simulink model "M002_SOFC_meca"  (R2021a)
settings: Solver=VariableStepAuto  StartTime=0.0  StopTime=1037  RelTol=1e-3
values from neighbouring files (symbols this model uses):
  p = SOFC_p    [M002_init_SOFC_meca.m]
  x0_SOFC = SOFC_init    [M002_init_SOFC_meca.m]
undefined symbols (not defined in the file or in its folder): nearst_p
settings Model: Creator=djoroya  LastModifiedBy=djoroya

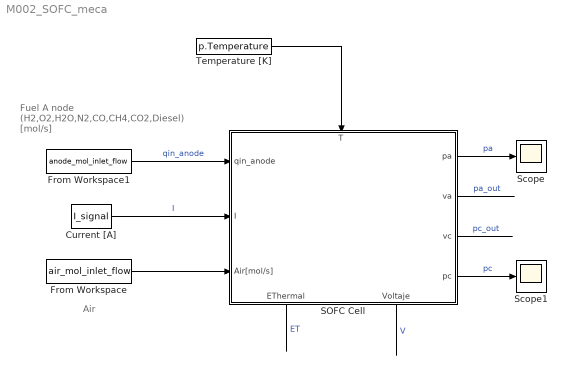
== system M002_SOFC_meca ==
  note: Fuel
      | A node
      | (H2,O2,H2O,N2,CO,CH4,CO2,Diesel)
      | [mol/s]
  note: Air
  Current [A] : FromWorkspace  VariableName=I_signal
  From Workspace : FromWorkspace  VariableName=air_mol_inlet_flow
  From Workspace1 : FromWorkspace  VariableName=anode_mol_inlet_flow
  SOFC Cell : Subsystem  mask{p=p, x0=x0_SOFC}
      mask prompts: p "params"
      settings: PortSchema="{\"entries\":[{\"content\":{\"sides\":[{\"content\":{\"connectorIds\":[\"In1\",\"In2\",\"In3\"]},\"type\":\"ConnectorPlacement.EquallySpacedRectSide\",\"uuid\":\"6cca8e4f-6db2-48de-a60a-b6fbc16877c6\"},{\"content\":{\"connectorIds\":[\"Out1\",\"Out2\",\"Out3\",\"Out4\"],\"side\":\"RIGHT\"},\"type\":\"ConnectorPlacement.EquallySpacedRectSide\",\"uuid\":\"c481f6d1-531d-4215-9ae0-5807376c0625\"},{\"content\":{\"connectorIds\":[\"In4\"],\"side\":\"TOP\"},\"type\":\"ConnectorPlacement.EquallySpacedRectSide\",\"uuid\":\"76720726-927e-4340-b17d-e33f4db2c782\"},{\"content\":{\"connectorIds\":[\"Out5\",\"Out6\"],\"side\":\"BOTTOM\"},\"type\":\"ConnectorPlacement.EquallySpacedRectSide\",\"uuid\":\"7ed108e3-6588-44d6-8f3d-9789ffe258a7\"}]},\"type\":\"ConnectorPlacement.EquallySpacedConnector\",\"uuid\":\"f9228f26-0840-43d6-932a-2fdb8a27bf20\"}],\"packageUris\":[\"http://schema.mathworks.com/mf0/Connector/R2020b\"],\"version\":\"1.0\"}"
  Scope : Scope
  Scope1 : Scope
  Temperature [K] : Constant  Value=p.Temperature
  wires:
  From Workspace1/1 -> SOFC Cell/1(qin_anode)  "qin_anode"
  Current [A]/1 -> SOFC Cell/2(I)  "I"
  Temperature [K]/1 -> SOFC Cell/4(T)
  From Workspace/1 -> SOFC Cell/3(Air[mol/s])
  SOFC Cell/1(pa) -> Scope/1  "pa"
  SOFC Cell/4(pc) -> Scope1/1  "pc"
  SOFC Cell/2(va) -> ?  "pa_out"
  SOFC Cell/3(vc) -> ?  "pc_out"
  SOFC Cell/5(EThermal) -> ?  "ET"
  SOFC Cell/6(Voltaje) -> ?  "V"

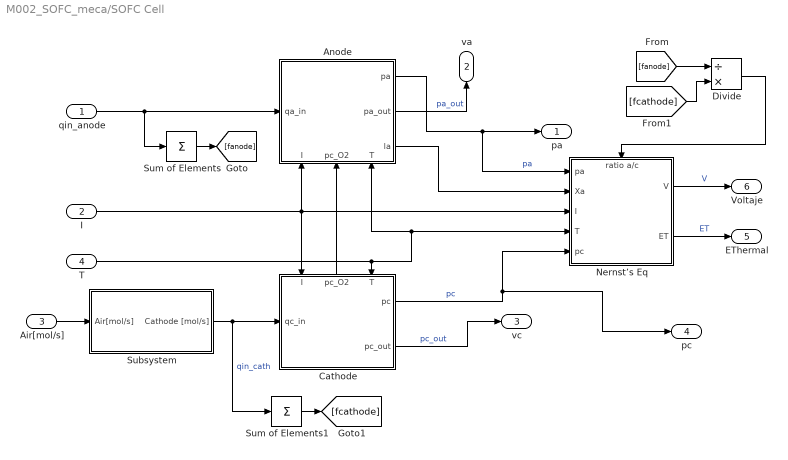
== system M002_SOFC_meca/SOFC Cell ==
  qin_anode : Inport
  I : Inport  Port=2
  Air[mol/s] : Inport  Port=3
  T : Inport  Port=4
  Anode : Subsystem
      settings: PortSchema="{\"entries\":[{\"content\":{\"sides\":[{\"content\":{\"connectorIds\":[\"In1\"]},\"type\":\"ConnectorPlacement.EquallySpacedRectSide\",\"uuid\":\"1d27f661-9cb9-482d-ac43-89e84d52643b\"},{\"content\":{\"connectorIds\":[\"Out1\",\"Out2\",\"Out3\"],\"side\":\"RIGHT\"},\"type\":\"ConnectorPlacement.EquallySpacedRectSide\",\"uuid\":\"62ac897d-5819-4e9c-a19f-e210851aefa2\"},{\"content\":{\"connectorIds\":[],\"side\":\"TOP\"},\"type\":\"ConnectorPlacement.EquallySpacedRectSide\",\"uuid\":\"1380e9d4-c5ac-42ce-b6fc-00336cc8edba\"},{\"content\":{\"connectorIds\":[\"In2\",\"In3\",\"In4\"],\"side\":\"BOTTOM\"},\"type\":\"ConnectorPlacement.EquallySpacedRectSide\",\"uuid\":\"0e36fd1a-38eb-48cb-8834-06d558b43614\"}]},\"type\":\"ConnectorPlacement.EquallySpacedConnector\",\"uuid\":\"79a72313-dbdc-4de5-b88f-787bafe984c7\"}],\"packageUris\":[\"http://schema.mathworks.com/mf0/Connector/R2020b\"],\"version\":\"1.0\"}"
  Cathode : Subsystem
      settings: PortSchema="{\"entries\":[{\"content\":{\"sides\":[{\"content\":{\"connectorIds\":[\"In1\"]},\"type\":\"ConnectorPlacement.EquallySpacedRectSide\",\"uuid\":\"1d27f661-9cb9-482d-ac43-89e84d52643b\"},{\"content\":{\"connectorIds\":[\"Out1\",\"Out2\"],\"side\":\"RIGHT\"},\"type\":\"ConnectorPlacement.EquallySpacedRectSide\",\"uuid\":\"62ac897d-5819-4e9c-a19f-e210851aefa2\"},{\"content\":{\"connectorIds\":[\"In2\",\"Out3\",\"In3\"],\"side\":\"TOP\"},\"type\":\"ConnectorPlacement.EquallySpacedRectSide\",\"uuid\":\"1380e9d4-c5ac-42ce-b6fc-00336cc8edba\"}]},\"type\":\"ConnectorPlacement.EquallySpacedConnector\",\"uuid\":\"79a72313-dbdc-4de5-b88f-787bafe984c7\"}],\"packageUris\":[\"http://schema.mathworks.com/mf0/Connector/R2020b\"],\"version\":\"1.0\"}"
  Divide : Product  Inputs=/*
  "Nernst’s Eq " : Subsystem
      settings: PortSchema="{\"entries\":[{\"content\":{\"sides\":[{\"content\":{\"connectorIds\":[\"In1\",\"In2\",\"In3\",\"In4\",\"In5\"]},\"type\":\"ConnectorPlacement.EquallySpacedRectSide\",\"uuid\":\"1b300774-e64d-4a8a-a2e9-ecdc71723fee\"},{\"content\":{\"connectorIds\":[\"Out1\",\"Out2\"],\"side\":\"RIGHT\"},\"type\":\"ConnectorPlacement.EquallySpacedRectSide\",\"uuid\":\"354a04f1-cc66-4a63-8c50-8080316e29e9\"},{\"content\":{\"connectorIds\":[\"In6\"],\"side\":\"TOP\"},\"type\":\"ConnectorPlacement.EquallySpacedRectSide\",\"uuid\":\"b48b7bda-dd37-468f-ab7d-ccd563a69f0b\"}]},\"type\":\"ConnectorPlacement.EquallySpacedConnector\",\"uuid\":\"ddfd4041-6e53-4893-9028-34e5ff9f82d6\"}],\"packageUris\":[\"http://schema.mathworks.com/mf0/Connector/R2020b\"],\"version\":\"1.0\"}"
  Subsystem : Subsystem
  Sum of Elements : Sum  Inputs=+
  Sum of Elements1 : Sum  Inputs=+
  pa : Outport
  va : Outport  Port=2
  vc : Outport  Port=3
  pc : Outport  Port=4
  EThermal : Outport  Port=5
  Voltaje : Outport  Port=6
  wires:
  Air[mol/s]/1 -> Subsystem/1(Air[mol/s])
  Anode/1(pa) -> pa/1, "Nernst’s Eq "/1(pa)  "pa"
  Anode/2(pa_out) -> va/1  "pa_out"
  Cathode/1(pc) -> pc/1, "Nernst’s Eq "/5(pc)  "pc"
  Subsystem/1(Cathode [mol/s]) -> Sum of Elements1/1, Cathode/1(qc_in)  "qin_cath"
  "Nernst’s Eq "/2(ET) -> EThermal/1  "ET"
  Cathode/3(pc_O2) -> Anode/3(pc_O2)
  Cathode/2(pc_out) -> vc/1  "pc_out"
  I/1 -> Cathode/2(I), "Nernst’s Eq "/3(I), Anode/2(I)
  T/1 -> "Nernst’s Eq "/4(T), Anode/4(T), Cathode/3(T)
  qin_anode/1 -> Anode/1(qa_in), Sum of Elements/1
  "Nernst’s Eq "/1(V) -> Voltaje/1  "V"
  Anode/3(la) -> "Nernst’s Eq "/2(Xa)
  Sum of Elements/1 -> [fanode]
  Sum of Elements1/1 -> [fcathode]
  [fanode] -> Divide/1
  [fcathode] -> Divide/2
  Divide/1 -> "Nernst’s Eq "/6(ratio a/c)

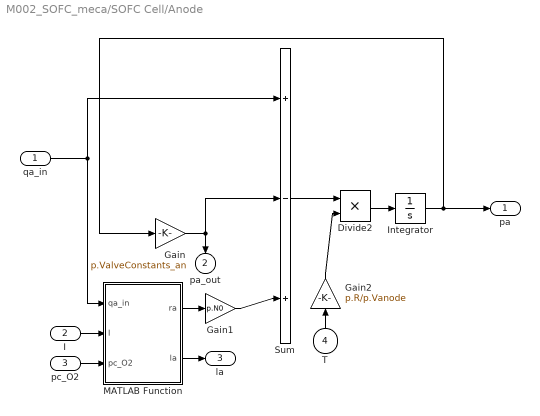
== system M002_SOFC_meca/SOFC Cell/Anode ==
  qa_in : Inport
  I : Inport  Port=2
  pc_O2 : Inport  Port=3
  T : Inport  Port=4
  Divide2 : Product  Inputs=**
  Gain : Gain  Gain=p.ValveConstants_an
  Gain1 : Gain  Gain=p.N0
  Gain2 : Gain  Gain=p.R/p.Vanode
  Integrator : Integrator  InitialCondition=x0_SOFC.pa
  MATLAB Function : MATLAB Function  TreatAsAtomicUnit=on
  Sum : Sum  Inputs=|+-+
  pa : Outport
  pa_out : Outport  Port=2
  la : Outport  Port=3
  wires:
  Sum/1 -> Divide2/1
  Integrator/1 -> pa/1, Gain/1
  Gain2/1 -> Divide2/2
  qa_in/1 -> Sum/1, MATLAB Function/1(qa_in)
  Divide2/1 -> Integrator/1
  Gain/1 -> pa_out/1, Sum/2
  I/1 -> MATLAB Function/2(I)
  T/1 -> Gain2/1
  MATLAB Function/2(la) -> la/1
  pc_O2/1 -> MATLAB Function/3(pc_O2)
  MATLAB Function/1(ra) -> Gain1/1
  Gain1/1 -> Sum/3

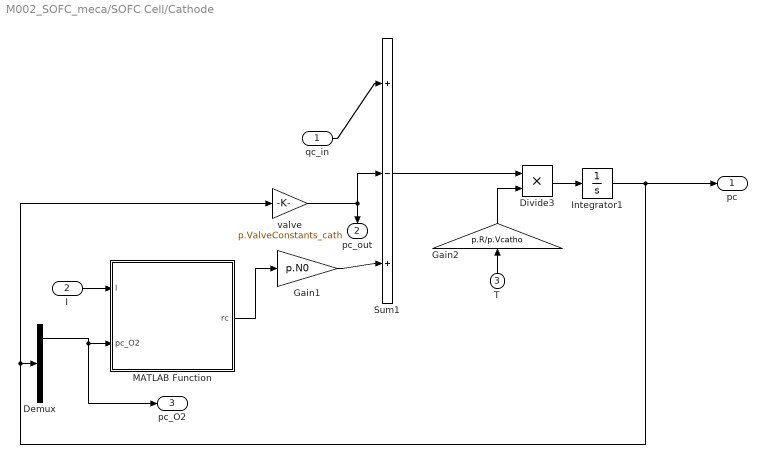
== system M002_SOFC_meca/SOFC Cell/Cathode ==
  qc_in : Inport
  I : Inport  Port=2
  T : Inport  Port=3
  Demux : Demux  Outputs=8
  Divide3 : Product  Inputs=**
  Gain1 : Gain  Gain=p.N0
  Gain2 : Gain  Gain=p.R/p.Vcatho
  Integrator1 : Integrator  InitialCondition=x0_SOFC.pc
  MATLAB Function : MATLAB Function  TreatAsAtomicUnit=on
  Sum1 : Sum  Inputs=|+-+
  valve : Gain  Gain=p.ValveConstants_cath
  pc : Outport
  pc_out : Outport  Port=2
  pc_O2 : Outport  Port=3
  wires:
  Sum1/1 -> Divide3/1
  Integrator1/1 -> valve/1, Demux/1, pc/1
  Divide3/1 -> Integrator1/1
  qc_in/1 -> Sum1/1
  Gain2/1 -> Divide3/2
  T/1 -> Gain2/1
  valve/1 -> pc_out/1, Sum1/2
  I/1 -> MATLAB Function/1(I)
  Demux/2 -> pc_O2/1, MATLAB Function/2(pc_O2)
  MATLAB Function/1(rc) -> Gain1/1
  Gain1/1 -> Sum1/3

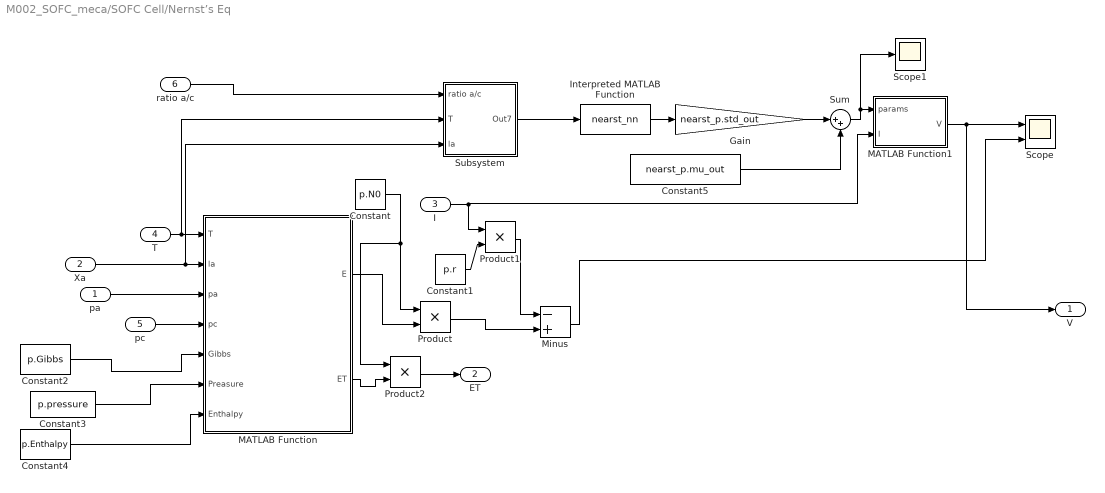
== system M002_SOFC_meca/SOFC Cell/Nernst’s Eq  ==
  pa : Inport
  Xa : Inport  Port=2
  I : Inport  Port=3
  T : Inport  Port=4
  pc : Inport  Port=5
  ratio a/c : Inport  Port=6
  Constant : Constant  Value=p.N0
  Constant1 : Constant  Value=p.r
  Constant2 : Constant  Value=p.Gibbs  OutDataTypeStr=Bus:slBus1
  Constant3 : Constant  Value=p.pressure
  Constant4 : Constant  Value=p.Enthalpy  OutDataTypeStr=Bus:slBus1
  Constant5 : Constant  Value=nearst_p.mu_out
  Gain : Gain  Gain=nearst_p.std_out
  Interpreted MATLAB Function : MATLABFcn  MATLABFcn=nearst_nn
  MATLAB Function : MATLAB Function  TreatAsAtomicUnit=on
  MATLAB Function1 : MATLAB Function  TreatAsAtomicUnit=on
  Minus : Sum  Inputs=-+
  Product : Product
  Product1 : Product
  Product2 : Product
  Scope : Scope  NumInputPorts=2
  Scope1 : Scope
  Subsystem : Subsystem
  Sum : Sum  Inputs=|++
  V : Outport
  ET : Outport  Port=2
  wires:
  MATLAB Function/1(E) -> Product/2
  Constant/1 -> Product2/1, Product/1
  I/1 -> Product1/1, MATLAB Function1/2(I)
  Constant1/1 -> Product1/2
  Product/1 -> Minus/2
  Minus/1 -> Scope/2
  Product1/1 -> Minus/1
  pa/1 -> MATLAB Function/3(pa)
  pc/1 -> MATLAB Function/4(pc)
  Constant2/1 -> MATLAB Function/5(Gibbs)
  T/1 -> Subsystem/2(T), MATLAB Function/1(T)
  Xa/1 -> Subsystem/3(la), MATLAB Function/2(la)
  Constant3/1 -> MATLAB Function/6(Preasure)
  Constant4/1 -> MATLAB Function/7(Enthalpy)
  Product2/1 -> ET/1
  MATLAB Function/2(ET) -> Product2/2
  ratio a/c/1 -> Subsystem/1(ratio a/c)
  Subsystem/1(Out7) -> Interpreted MATLAB Function/1
  Interpreted MATLAB Function/1 -> Gain/1
  Gain/1 -> Sum/1
  Constant5/1 -> Sum/2
  Sum/1 -> Scope1/1, MATLAB Function1/1(params)
  MATLAB Function1/1(V) -> V/1, Scope/1

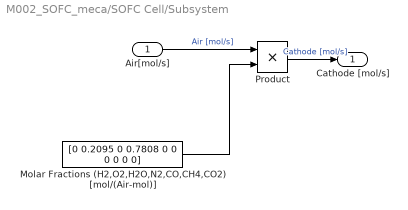
== system M002_SOFC_meca/SOFC Cell/Subsystem ==
  Air[mol/s] : Inport
  Molar Fractions (H2,O2,H2O,N2,CO,CH4,CO2) [mol/(Air-mol)] : Constant  Value=[0 0.2095 0 0.7808 0 0 0 0 0 0]
  Product : Product
  Cathode [mol/s] : Outport
  wires:
  Air[mol/s]/1 -> Product/1  "Air [mol/s]"
  Product/1 -> Cathode [mol/s]/1  "Cathode [mol/s]"
  Molar Fractions (H2,O2,H2O,N2,CO,CH4,CO2) [mol/(Air-mol)]/1 -> Product/2

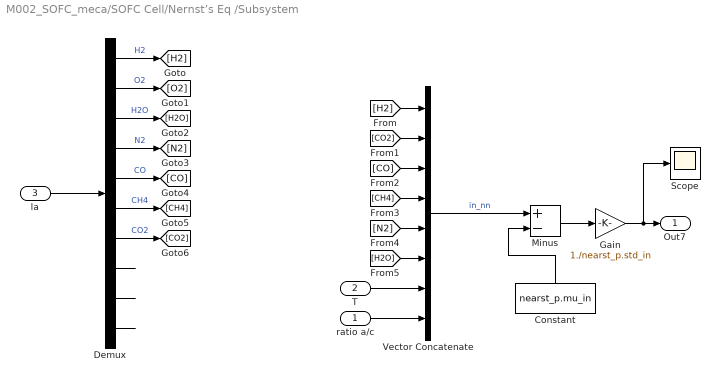
== system M002_SOFC_meca/SOFC Cell/Nernst’s Eq /Subsystem ==
  ratio a/c : Inport
  T : Inport  Port=2
  la : Inport  Port=3
  Constant : Constant  Value=nearst_p.mu_in
  Demux : Demux  Outputs=10
  Gain : Gain  Gain=1./nearst_p.std_in
  Minus : Sum  Inputs=+-
  Scope : Scope
  Vector Concatenate : Concatenate  NumInputs=8
  Out7 : Outport
  wires:
  Demux/7 -> [CO2]  "CO2"
  la/1 -> Demux/1
  Demux/3 -> [H2O]  "H2O"
  Demux/1 -> [H2]  "H2"
  Demux/8 -> ?
  Demux/2 -> [O2]  "O2"
  Demux/10 -> ?
  Demux/9 -> ?
  Demux/5 -> [CO]  "CO"
  Demux/4 -> [N2]  "N2"
  Demux/6 -> [CH4]  "CH4"
  ratio a/c/1 -> Vector Concatenate/8
  T/1 -> Vector Concatenate/7
  [H2] -> Vector Concatenate/1
  [CO2] -> Vector Concatenate/2
  [CO] -> Vector Concatenate/3
  [CH4] -> Vector Concatenate/4
  [N2] -> Vector Concatenate/5
  [H2O] -> Vector Concatenate/6
  Vector Concatenate/1 -> Minus/1  "in_nn"
  Constant/1 -> Minus/2
  Minus/1 -> Gain/1
  Gain/1 -> Scope/1, Out7/1

== matlab function M002_SOFC_meca/SOFC Cell/Cathode/MATLAB Function ==
  data: rc output; I input; pc_O2 input
function rc = fcn(I,pc_O2)

%l = qc_in/sum(qc_in);

% l_H2  = l(1);
% l_O2  = l(2);
% l_H2O = l(3);
% l_N2  = l(4);
% l_CO  = l(5);
% l_CH4 = l(6);
% l_CO2 = l(7);
%
% alpha_H_2 = l_H2;
% alpha_CO  = l_CO;
% alpha_CH4 = l_CH4;
% alpha_O2  = 0.5*(l_H2+l_CO+4*l_CH4);
% beta_H2O  = l_H2 + 2*l_CH4;
% beta_CO2  = l_CO + 2*l_CH4;
%
F = 96485.3329; 

% r_H2  = -alpha_H_2*I;
% r_CO  = -alpha_CO*I;
% r_CH4 = -alpha_CH4*I;
% r_H20 = beta_H2O*I;
% r_CO2 = beta_CO2*I;
if pc_O2 <= 0
    r_O2  = 0;
else
    r_O2  = I/(4*F);
end

rc = [0 -r_O2 0 0 0 0 0 0 0 0]';

== matlab function M002_SOFC_meca/SOFC Cell/Anode/MATLAB Function ==
  data: qa_in input; ra output; I input; la output; pc_O2 input
function [ra,la] = fcn(qa_in,I,pc_O2)

la = qa_in/sum(qa_in);

l_H2  = la(1);
%l_O2  = l(2);
%l_H2O = l(3);
%l_N2  = l(4);
l_CO  = la(5);
l_CH4 = la(6);
%l_CO2 = l(7);
%
alpha_H2 = l_H2;
alpha_CO  = l_CO;
alpha_CH4 = l_CH4;
%alpha_O2  = 0.5*(l_H2+l_CO+4*l_CH4);
beta_H2O  = l_H2 + 2*l_CH4;
beta_CO2  = l_CO + l_CH4;
%
F = 96485.3329; 
ne = 2*(l_H2 + l_CO + 4*l_CH4);
I = I/(F*ne);

r_H2  = -alpha_H2*I;
r_CO  = -alpha_CO*I;
r_CH4 = -alpha_CH4*I;
r_H20 = beta_H2O*I;
r_CO2 = beta_CO2*I;
%
ra = [r_H2 0 r_H20 0 r_CO r_CH4 r_CO2 0 0 0]';

if pc_O2 <= 0
    ra  = 0*ra;
end

== matlab function M002_SOFC_meca/SOFC Cell/Nernst’s Eq /MATLAB Function ==
  data: T input; la input; pa input; E output; pc input; Gibbs input; Preasure input; Enthalpy input; ET output
function [E,ET]= fcn(T, la,pa,pc,Gibbs,Preasure, Enthalpy)
%

l_H2  = la(1);
l_CO  = la(5);
l_CH4 = la(6);
%
alpha_H2 = l_H2;
alpha_CO  = l_CO;
alpha_CH4 = l_CH4;
alpha_O2  = 0.5*( l_H2 + l_CO + 4*l_CH4);
beta_H2O  = l_H2 + 2*l_CH4;
beta_CO2  = l_CO + l_CH4;

%
pa_H2 = pa(1);
pa_O2 = pa(2);
pa_H2O= pa(3);
pa_CO = pa(5);
pa_CH4= pa(6);
pa_CO2= pa(7);
%
pc_H2 = pc(1);
pc_O2 = pc(2);
pc_H2O= pc(3);
pc_N2 = pc(4);
pc_CO = pc(5);
pc_CH4= pc(6);
pc_CO2= pc(7);
%% 
F = 96485.3329; 
ne = 2*(l_H2 + l_CO + 4*l_CH4);
%%
G = alpha_H2*Gibbs.H2 + ...
    alpha_CO*Gibbs.CO + ...
    alpha_CH4*Gibbs.CH4 + ...
    alpha_O2*Gibbs.O2 + ...
    - beta_H2O*Gibbs.H2O + ...
    - beta_CO2*Gibbs.CO2;
%%
E0 = G/(F*ne); 

%%
R = 8.31446261815324;

ab =    [alpha_H2, ...
         alpha_CO, ...
         alpha_CH4, ...
         alpha_O2,  ...
         -beta_H2O, ...
         -beta_CO2];
     
pa_ab = [pa_H2, ...
         pa_CO, ...
         pa_CH4, ...
         pc_O2,  ...
         pa_H2O, ...
         pa_CO2];
     
log_ab = 0*ab;
iter = 0;
for ipa_ab = pa_ab
    iter = iter + 1;
    if ipa_ab > 0
       log_ab(iter) =  log(ipa_ab/Preasure);
    end
end

E = E0 + ((R*T)/(ne*F))*( sum(log_ab.*ab) );

%%
H = alpha_H2*Enthalpy.H2 + ...
    alpha_CO*Enthalpy.CO + ...
    alpha_CH4*Enthalpy.CH4 + ...
    alpha_O2*Enthalpy.O2 + ...
    - beta_H2O*Enthalpy.H2O + ...
    - beta_CO2*Enthalpy.CO2;
ET = H/(ne*F);
%

== matlab function M002_SOFC_meca/SOFC Cell/Nernst’s Eq /MATLAB Function1 ==
  data: params input; V output; I input
function V = fcn(params, I)

A_esti =  params(1);
E0_esti =  params(2);
R_esti =  params(3);

m = 0.5355;
n = 0.0313;


V = E0_esti - I.*R_esti - A_esti*log(I) - m*exp(n*I);
